simulink model "eha_model_w_iir"  (R2015b)
settings: Solver=ode4  StartTime=0.0  StopTime=20  FixedStep=0.01  RelTol=1e-3
values from neighbouring files (symbols this model uses):
  A = [ 1 0.001 0; 0 1 0.001; -557.02 -28.616 0.9418]    [eha_w_iir_filter.m]
  B = [0 0 557.02]'    [eha_w_iir_filter.m]
  C = H    [eha_w_iir_filter.m]
  x0 = [0 0 0]'    [eha_w_iir_filter.m]
settings Model: Creator=mathi  LastModifiedBy=Nicholas

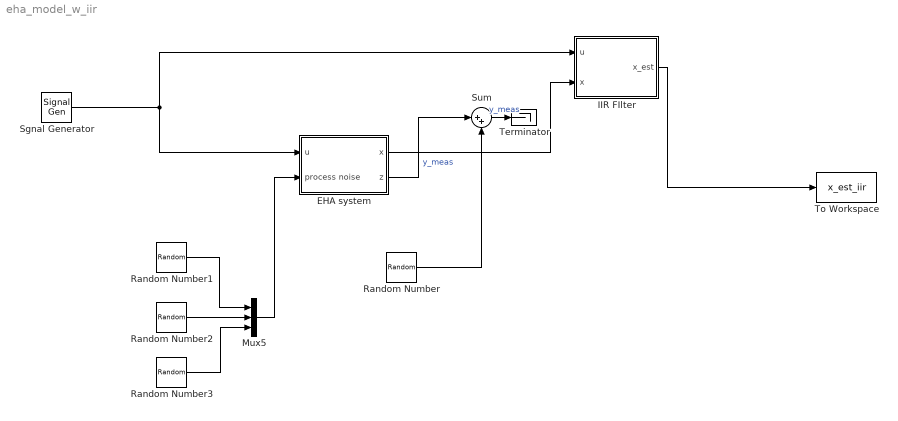
== system eha_model_w_iir ==
  EHA system : Subsystem
  IIR FIlter : Subsystem
  Mux5 : Mux  Inputs=3
  Random Number : RandomNumber  Variance=0.1  SampleTime=0.01
  Random Number1 : RandomNumber  Variance=0.001  SampleTime=0.01
  Random Number2 : RandomNumber  SampleTime=0.01
  Random Number3 : RandomNumber  Variance=10  SampleTime=0.01
  Sgnal Generator : SignalGenerator  WaveForm=square  Units=rad/sec
  Sum : Sum  Inputs=|++
  Terminator : Terminator
  To Workspace : ToWorkspace  VariableName=x_est_iir  SaveFormat=Timeseries  SampleTime=-1
  wires:
  Sgnal Generator/1 -> IIR FIlter/1(u), EHA system/1(u)
  EHA system/2(z) -> Sum/1  "y_meas"
  Random Number/1 -> Sum/2
  EHA system/1(x) -> IIR FIlter/2(x)
  Random Number1/1 -> Mux5/1
  Random Number2/1 -> Mux5/2
  Random Number3/1 -> Mux5/3
  Mux5/1 -> EHA system/2(process noise)
  Sum/1 -> Terminator/1  "y_meas"
  IIR FIlter/1(x_est) -> To Workspace/1

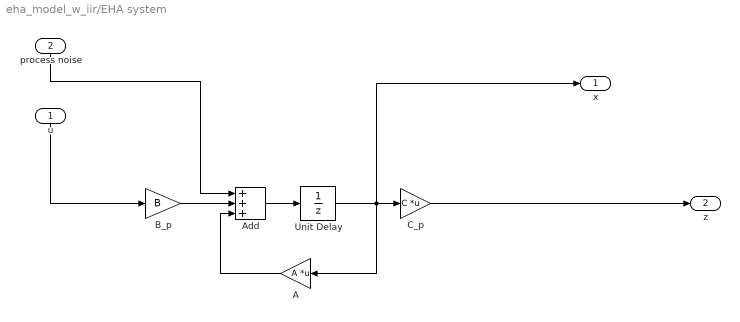
== system eha_model_w_iir/EHA system ==
  u : Inport
  process noise : Inport  Port=2
  A : Gain  Gain=A  Multiplication=Matrix(K*u)
  Add : Sum  Inputs=+++
  B_p : Gain  Gain=B
  C_p : Gain  Gain=C  Multiplication=Matrix(K*u)
  Unit Delay : UnitDelay  InitialCondition=x0  SampleTime=-1
  x : Outport
  z : Outport  Port=2
  wires:
  Unit Delay/1 -> C_p/1, x/1, A/1
  C_p/1 -> z/1
  u/1 -> B_p/1
  Add/1 -> Unit Delay/1
  B_p/1 -> Add/2
  A/1 -> Add/3
  process noise/1 -> Add/1

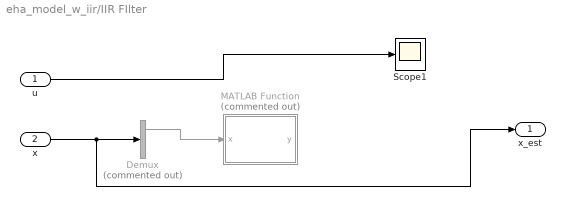
== system eha_model_w_iir/IIR FIlter ==
  u : Inport
  x : Inport  Port=2
  Demux : Demux  Commented=on  Outputs=3
  MATLAB Function : MATLAB Function  Commented=on  TreatAsAtomicUnit=on
  Scope1 : Scope
  x_est : Outport
  wires:
  u/1 -> Scope1/1
  x/1 -> x_est/1, Demux/1
  Demux/1 -> MATLAB Function/1(x)

== matlab function eha_model_w_iir/IIR FIlter/MATLAB Function ==
  data: x input; y output
function y = fcn(x)
%#codegen
N = [0.2929 0.5858 0.2929];
D = [1 0 0.1716];
% H = tf(num,den,0.01);
% [A,B,C,D] = tf2ss(N,D)
% [N,D] = butter(5, 0.5, 'low');

y = filter(N, D, x);
